simulink model "DFIG_DPC_SVM"  (R2023b)
settings: Solver=ode4  StartTime=0.0  StopTime=1  FixedStep=5e-6  MaxStep=5e-6  RelTol=1e-3
libraries: spspowerguiLib x1
settings Model: Creator=Y  LastModifiedBy=Y

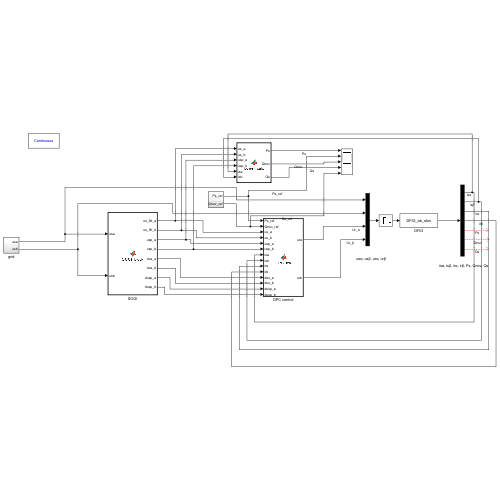
[thumbnail: Simulink's stored preview of the top-level diagram]
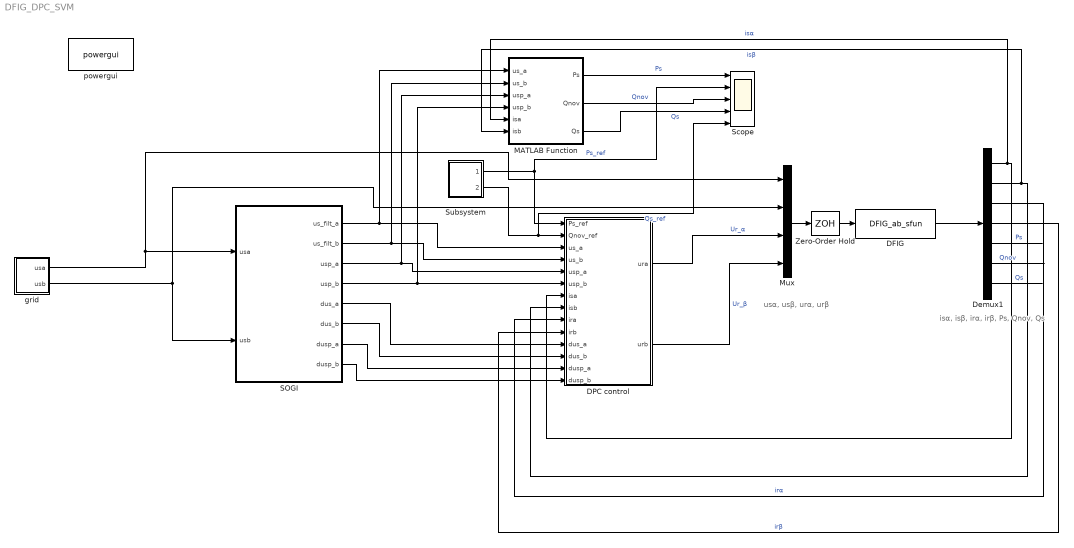
== system DFIG_DPC_SVM ==
  note: isα, isβ, irα, irβ, Ps, Qnov, Qs
  note: usα, usβ, urα, urβ
  DFIG : S-Function  FunctionName=DFIG_ab_sfun  SFunctionDeploymentMode=off  EnableBusSupport=off
  DPC control : MATLAB Function  TreatAsAtomicUnit=on
  Demux1 : Demux  Outputs=7
  MATLAB Function : MATLAB Function  TreatAsAtomicUnit=on
  Mux : Mux
  SOGI : MATLAB Function  TreatAsAtomicUnit=on
  Scope : Scope  NumInputPorts=5
  Subsystem : Subsystem
  Zero-Order Hold : ZeroOrderHold  SampleTime=-1
  grid : Subsystem
  powergui : spspowerguiLib/powergui  Priority=1  SimulationMode=Continuous  SampleTime=50e-6  frequency=60  Iterations=50  frequencyindice=50  Pbase=100e6  ErrMax=1e-4  UnitsV=kV  UnitsW=MW  buscounter=0  FunctionMessages=off  echomessages=off  EnableUseOfTLC=off  CurrentSourceSwitches=off  DisableSnubberDevices=off  DisableRonSwitches=off  DisableVfSwitches=off  DisplayEquations=off  AutomaticDiscreteSolvers=off  SolverType=Tustin/Backward Euler (TBE)  Interpol=off  ExternalGateDelay=off  methode=off  Ts=100  x0status=blocks  SPID=on  SwTol=0  HookPort=off  NonlinearTolerance=1e-4  nMaxIteration=100  ContinueOnMaxIteration=off  RestoreLinks=warning  ResistiveCurrentMeasurement=off  Frange=[0:2:500]  Ylog=off  Xlog=on  ShowGrid=off  save=off  variable=ZData  structure=0  ZoomFFT=off  StartTime=0.0  cycles=1  DisplayStyle=1  fundamental=60  FreqAxis=off  MaxFrequency=1000  frequencyindicesteady=1  RmsSteady=1  display=off
  wires:
  DPC control/1(ura) -> Mux/3  "Ur_α"
  DPC control/2(urb) -> Mux/4  "Ur_β"
  Mux/1 -> Zero-Order Hold/1
  DFIG/1 -> Demux1/1
  Demux1/1 -> MATLAB Function/5(isa), DPC control/7(isa)  "isα"
  SOGI/1(us_filt_a) -> MATLAB Function/1(us_a), DPC control/3(us_a)
  SOGI/2(us_filt_b) -> MATLAB Function/2(us_b), DPC control/4(us_b)
  SOGI/3(usp_a) -> MATLAB Function/3(usp_a), DPC control/5(usp_a)
  SOGI/4(usp_b) -> MATLAB Function/4(usp_b), DPC control/6(usp_b)
  Demux1/2 -> MATLAB Function/6(isb), DPC control/8(isb)  "isβ"
  Demux1/3 -> DPC control/9(ira)  "irα"
  Demux1/4 -> DPC control/10(irb)  "irβ"
  Demux1/5 -> ?  "Ps"
  Demux1/6 -> ?  "Qnov"
  Demux1/7 -> ?  "Qs"
  SOGI/5(dus_a) -> DPC control/11(dus_a)
  SOGI/6(dus_b) -> DPC control/12(dus_b)
  SOGI/7(dusp_a) -> DPC control/13(dusp_a)
  SOGI/8(dusp_b) -> DPC control/14(dusp_b)
  Subsystem/2(Qnov_ref) -> Scope/5, DPC control/2(Qnov_ref)  "Qs_ref"
  MATLAB Function/1(Ps) -> Scope/1  "Ps"
  Subsystem/1(Ps_ref) -> Scope/2, DPC control/1(Ps_ref)  "Ps_ref"
  MATLAB Function/2(Qnov) -> Scope/3  "Qnov"
  MATLAB Function/3(Qs) -> Scope/4  "Qs"
  Zero-Order Hold/1 -> DFIG/1
  grid/2(usb) -> Mux/2, SOGI/2(usb)
  grid/1(usa) -> Mux/1, SOGI/1(usa)

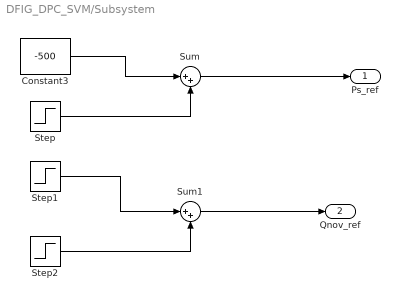
== system DFIG_DPC_SVM/Subsystem ==
  Constant3 : Constant  Value=-500
  Step : Step  Time=0.3  After=-500  SampleTime=0
  Step1 : Step  Time=0.3  After=-300  SampleTime=0
  Step2 : Step  Time=0.5  After=300  SampleTime=0
  Sum : Sum  Inputs=|++
  Sum1 : Sum  Inputs=|++
  Ps_ref : Outport
  Qnov_ref : Outport  Port=2
  wires:
  Step1/1 -> Sum1/1
  Step/1 -> Sum/2
  Step2/1 -> Sum1/2
  Constant3/1 -> Sum/1
  Sum/1 -> Ps_ref/1
  Sum1/1 -> Qnov_ref/1

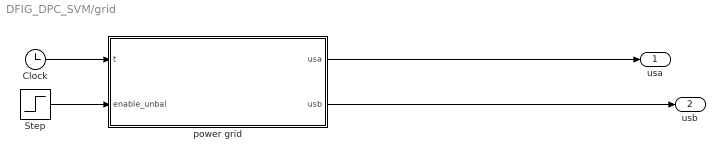
== system DFIG_DPC_SVM/grid ==
  Clock : Clock
  Step : Step  Time=0.5  SampleTime=0
  power grid : MATLAB Function  TreatAsAtomicUnit=on
  usa : Outport
  usb : Outport  Port=2
  wires:
  power grid/1(usa) -> usa/1
  power grid/2(usb) -> usb/1
  Clock/1 -> power grid/1(t)
  Step/1 -> power grid/2(enable_unbal)

== matlab function DFIG_DPC_SVM/SOGI ==
  settings: updateMethod=DISCRETE  sampleTime=5e-6
  data: usa input; us_filt_a output; usb input; us_filt_b output; usp_a output; usp_b output; dus_a output; dus_b output; dusp_a output; dusp_b output
function [us_filt_a, us_filt_b, usp_a, usp_b, ...
          dus_a, dus_b, dusp_a, dusp_b] = SOGI_block(usa, usb)
% 双路 SOGI：提取滤波电压 + 正交电压 + 电压导数
% us_filt: 滤波后的基波电压
% usp: 正交电压（滞后 90°）
% dus, dusp: 对应的导数

k = sqrt(2);      % SOGI 增益
w = 2*pi*50;       % 谐振频率
Tsc = 5e-6;      % 控制周期（= 此块的采样率）

persistent xa xb
if isempty(xa)
    xa = [usa; 0];   % [v'; qv'] for α  xa(1)  SOGI 的滤波输出，即输入信号经过带通滤波后的结果，初始化为 usa（当前输入值），让滤波器从接近真实值的地方开始，减少启动暂态
    xb = [usb; 0];   % [v'; qv'] for β  xa(2)  SOGI 的正交输出，即滞后 90° 的信号。初始化为 0
end

% α 轴 SOGI
err_a = usa - xa(1);
dxa1 = k*w*err_a - w*xa(2);
dxa2 = w*xa(1);
xa = xa + Tsc * [dxa1; dxa2];

% β 轴 SOGI
err_b = usb - xb(1);
dxb1 = k*w*err_b - w*xb(2);
dxb2 = w*xb(1);
xb = xb + Tsc * [dxb1; dxb2];

% 输出
us_filt_a = xa(1);    % 滤波 usα
us_filt_b = xb(1);    % 滤波 usβ
usp_a = xa(2);        % us'α（正交）
usp_b = xb(2);        % us'β（正交）

% 电压导数（从 SOGI 状态方程直接获取）
dus_a = k*w*(usa - xa(1)) - w*xa(2);
dus_b = k*w*(usb - xb(1)) - w*xb(2);
dusp_a = w*xa(1);
dusp_b = w*xb(1);
%% 修正：在更新前保存导数
% dus_a = dxa1;    % 当前步导数
% dus_b = dxb1;
% dusp_a = dxa2;
% dusp_b = dxb2;
end

== matlab function DFIG_DPC_SVM/DPC control ==
  settings: updateMethod=DISCRETE  sampleTime=200e-6
  data: Ps_ref input; ura output; Qnov_ref input; us_a input; us_b input; usp_a input; usp_b input; isa input; isb input; ira input; irb input; dus_a input; dus_b input; dusp_a input; dusp_b input; urb output
function [ura, urb] = DPC_fcn(Ps_ref, Qnov_ref, ...
    us_a, us_b, usp_a, usp_b, ...
    isa, isb, ira, irb, ...
    dus_a, dus_b, dusp_a, dusp_b)
% DPC-SVM 死区控制律（论文式 36）

% 参数
Rs = 2.3; Rr = 1.83;
Ls = 0.2413; Lr = 0.2413; Lm = 0.2258;
Np = 2; Vdc = 400;
D = Ls*Lr - Lm^2;
lam = 1/D;           % λ
wm = 188.5;
wr = Np * wm;
Tsc = 200e-6;

% 转子磁链估算
psi_ra = Lr*ira + Lm*isa;
psi_rb = Lr*irb + Lm*isb;

% 当前功率
Ps   = 1.5 * (us_a*isa + us_b*isb);
Qnov = 1.5 * (usp_a*isa + usp_b*isb);

% 功率变化率要求
dPs_req   = (Ps_ref - Ps) / Tsc;
dQnov_req = (Qnov_ref - Qnov) / Tsc;

% 前馈项 fp
us_dot_is = us_a*isa + us_b*isb;
us_dot_ir = us_a*ira + us_b*irb;
us_sq = us_a^2 + us_b^2;
us_x_pr = us_a*psi_rb - us_b*psi_ra;
fp = 1.5*(lam*Lr*(us_sq - Rs*us_dot_is) ...
   + lam*Lm*(Rr*us_dot_ir + wr*us_x_pr) ...
   + isa*dus_a + isb*dus_b);

% 前馈项 fq
usp_dot_us = usp_a*us_a + usp_b*us_b;
usp_dot_is = usp_a*isa + usp_b*isb;
usp_dot_ir = usp_a*ira + usp_b*irb;
usp_x_pr = usp_a*psi_rb - usp_b*psi_ra;
fq = 1.5*(lam*Lr*(usp_dot_us - Rs*usp_dot_is) ...
   + lam*Lm*(Rr*usp_dot_ir + wr*usp_x_pr) ...
   + isa*dusp_a + isb*dusp_b);

% 行列式
sigma_det = us_a*usp_b - us_b*usp_a;

% 死区控制律
coeff = -2/(3*lam*Lm);
rhs1 = dPs_req - fp;
rhs2 = dQnov_req - fq;

if abs(sigma_det) < 1e-6%当电压太小（启动阶段）或 us​ 与 us′​ 几乎平行时，M 不可逆，此时输出零电压避免除零。
    ura = 0;
    urb = 0;
else
    ura = coeff/sigma_det * ( usp_b*rhs1 - us_b*rhs2);
    urb = coeff/sigma_det * (-usp_a*rhs1 + us_a*rhs2);
end

% 电压限幅
Vr_max = Vdc / sqrt(3);
ur_mag = sqrt(ura^2 + urb^2);
if ur_mag > Vr_max
    ura = ura * Vr_max / ur_mag;
    urb = urb * Vr_max / ur_mag;
end
end

== matlab function DFIG_DPC_SVM/MATLAB Function ==
  data: us_a input; Ps output; us_b input; usp_a input; usp_b input; isa input; isb input; Qnov output; Qs output
function [Ps, Qnov, Qs] = power_calc(us_a, us_b, usp_a, usp_b, isa, isb)
Ps   = 1.5 * (us_a*isa + us_b*isb);
Qnov = 1.5 * (usp_a*isa + usp_b*isb);
Qs   = 1.5 * (us_b*isa - us_a*isb);
end

== matlab function DFIG_DPC_SVM/grid/power grid ==
  data: t input; usa output; enable_unbal input; usb output
function [usa, usb] = grid_voltage_unbal(t, enable_unbal)
% 电网电压（Clarke 变换后的 αβ 分量）
% enable_unbal: 0=平衡, 1=A 相跌至 70%

Vs = 380*sqrt(2)/sqrt(3);  % 相电压峰值 ≈ 311V
ws = 2*pi*50;

if enable_unbal > 0.5
    va = 0.7 * Vs * cos(ws*t);
else
    va = Vs * cos(ws*t);
end
vb = Vs * cos(ws*t - 2*pi/3);
vc = Vs * cos(ws*t + 2*pi/3);

% Clarke 变换（等幅值）
usa = 2/3 * (va - 0.5*vb - 0.5*vc);
usb = (vb - vc) / sqrt(3);
end
